simulink model "Template_v3_08_2020a"  (R2020a)
settings: Solver=FixedStepAuto  StartTime=0.0  StopTime=tsim  FixedStep=baseRate  RelTol=1e-3  EnableMultiTasking=on
values from neighbouring files (symbols this model uses):
  baseRate = 0.05    [Run_Initializer.m]
  drop_states_ARM = [ pi/2, pi/2, 0]    [Run_Initializer.m]
  drop_states_BLACK = [ xLength/2, yLength/2, 0]    [Run_Initializer.m]
  drop_states_BLUE = [ xLength/2-0.5; yLength/2; 0]    [Run_Initializer.m]
  drop_states_RED = [ xLength/2+0.5, yLength/2, pi]    [Run_Initializer.m]
  F_Black_X_nominal = 0.2196    [Run_Initializer.m]
  F_Black_Y_nominal = 0.2825    [Run_Initializer.m]
  F_Blue_X_nominal = 0.2196    [Run_Initializer.m]
  F_Blue_Y_nominal = 0.2825    [Run_Initializer.m]
  F_red_X_nominal = 0.2196    [Run_Initializer.m]
  F_red_Y_nominal = 0.2825    [Run_Initializer.m]
  F_thrusters_BLACK = [F_Black_X_nominal; F_Black_X_nominal;                             F_Black_Y_nominal; F_Black_Y_nominal; F_Black_X_nominal;                              F_Black_X_nominal; F_Black_Y_nominal; F_Black_Y_nominal]    [Run_Initializer.m]
  F_thrusters_BLUE = [F_Blue_X_nominal; F_Blue_X_nominal;                             F_Blue_Y_nominal; F_Blue_Y_nominal; F_Blue_X_nominal;                              F_Blue_X_nominal; F_Blue_Y_nominal; F_Blue_Y_nominal]    [Run_Initializer.m]
  F_thrusters_RED = [F_red_X_nominal; F_red_X_nominal;                             F_red_Y_nominal; F_red_Y_nominal; F_red_X_nominal;                              F_red_X_nominal; F_red_Y_nominal; F_red_Y_nominal]    [Run_Initializer.m]
  Gamma1 = 0.0025    [Run_Initializer.m]
  Gamma2 = 100    [Run_Initializer.m]
  Gamma3 = 10    [Run_Initializer.m]
  Gamma4 = 0.001    [Run_Initializer.m]
  Gamma5 = 100    [Run_Initializer.m]
  Gamma6 = 0.001    [Run_Initializer.m]
  home_states_BLACK = [ xLength/2; yLength/2; 0]    [Run_Initializer.m]
  home_states_BLUE = [ xLength/2-0.9; yLength/2; 0]    [Run_Initializer.m]
  home_states_RED = [ xLength/2+0.9; yLength/2; pi]    [Run_Initializer.m]
  init_states_BLACK = [ xLength/2; yLength/2; 0]    [Run_Initializer.m]
  init_states_BLUE = [ xLength/2-0.9; yLength/2; 0]    [Run_Initializer.m]
  init_states_RED = [ xLength/2+0.9; yLength/2; pi]    [Run_Initializer.m]
  Kd_elarm = 0.05    [Run_Initializer.m]
  Kd_sharm = 0.05    [Run_Initializer.m]
  Kd_tb = 0.4    [Run_Initializer.m]
  Kd_tblue = 0.4    [Run_Initializer.m]
  Kd_tr = 0.4    [Run_Initializer.m]
  Kd_wrarm = 0.005    [Run_Initializer.m]
  Kd_xb = 8    [Run_Initializer.m]
  Kd_xblue = 8    [Run_Initializer.m]
  Kd_xr = 8    [Run_Initializer.m]
  Kd_yb = 8    [Run_Initializer.m]
  Kd_yblue = 8    [Run_Initializer.m]
  Kd_yr = 8    [Run_Initializer.m]
  Kp = [0.08 0 0 ... (first row only)    [Run_Initializer.m]
  Kp_elarm = 0.08    [Run_Initializer.m]
  Kp_sharm = 0.15    [Run_Initializer.m]
  Kp_tb = 0.1    [Run_Initializer.m]
  Kp_tblue = 0.1    [Run_Initializer.m]
  Kp_tr = 0.1    [Run_Initializer.m]
  Kp_wrarm = 0.007    [Run_Initializer.m]
  Kp_xb = 2    [Run_Initializer.m]
  Kp_xblue = 2    [Run_Initializer.m]
  Kp_xr = 2    [Run_Initializer.m]
  Kp_yb = 2    [Run_Initializer.m]
  Kp_yblue = 2    [Run_Initializer.m]
  Kp_yr = 2    [Run_Initializer.m]
  Kv = [0.05 0 0 ... (first row only)    [Run_Initializer.m]
  noise_variance_BLACK = 0    [Run_Initializer.m]
  noise_variance_BLUE = 0    [Run_Initializer.m]
  noise_variance_RED = 0    [Run_Initializer.m]
  Phase0_End = Phase0_Duration    (= 10)    [Run_Initializer.m]
  Phase1_End = Phase0_Duration + Phase1_Duration    (= 15)    [Run_Initializer.m]
  Phase2_End = Phase0_Duration + Phase1_Duration +                                   Phase2_Duration    (= 35)    [Run_Initializer.m]
  Phase3_End = Phase0_Duration + Phase1_Duration +                                   Phase2_Duration + Phase3_Duration    (= 550)    [Run_Initializer.m]
  Phase3_SubPhase1_End = Phase2_End + Phase3_SubPhase1_Duration    (= 155)    [Run_Initializer.m]
  Phase3_SubPhase2_End = Phase2_End + Phase3_SubPhase1_Duration +                                   Phase3_SubPhase2_Duration    (= 165)    [Run_Initializer.m]
  Phase3_SubPhase3_End = Phase2_End + Phase3_SubPhase1_Duration +                                   Phase3_SubPhase2_Duration +                                  Phase3_SubPhase3_Duration    (= 195)    [Run_Initializer.m]
  Phase3_SubPhase4_End = Phase2_End + Phase3_SubPhase1_Duration +                                   Phase3_SubPhase2_Duration +                                  Phase3_SubPhase3_Duration +                                  Phase3_SubPhase4_Duration    [Run_Initializer.m]
  Phase4_End = Phase0_Duration + Phase1_Duration +                                   Phase2_Duration + Phase3_Duration +                                   Phase4_Duration    (= 670)    [Run_Initializer.m]
  Phase5_End = Phase0_Duration + Phase1_Duration +                                   Phase2_Duration + Phase3_Duration +                                   Phase4_Duration + Phase5_Duration    (= 690)    [Run_Initializer.m]
  thruster_dist2CG_BLACK = [83.42;-52.58;55.94;-60.05;54.08;-53.92;77.06;-55.94]    [Run_Initializer.m]
  thruster_dist2CG_BLUE = [73.54;-64.46;81.39;-60.11;64.46;-65.94;54.61;-74.39]    [Run_Initializer.m]
  thruster_dist2CG_RED = [49.92;-78.08;70.46;-63.54;81.08;-50.42;57.44;-75.96]    [Run_Initializer.m]
  Tz_lim_elarm = .1    (= 0.1)    [Run_Initializer.m]
  Tz_lim_sharm = .1    (= 0.1)    [Run_Initializer.m]
  Tz_lim_wrarm = .1    (= 0.1)    [Run_Initializer.m]
  xLength = 3.51155    [Run_Initializer.m]
  yLength = 2.41935    [Run_Initializer.m]
undefined symbols (not defined in the file or in its folder): DiscIntNeverNeededParam, model_param, platformSelection, serverRate, simMode
libraries: dspstat3 x18, raspberrypiBasiclib x10, embdlinuxlib x7, MainLibrary x6, dspsigops x6, simulink x6, mspfiltlib x3, dsparch4 x3, sensehatlib x1
(part 14 of 14)

== matlab function Template_v3_08_2020a/Phase #4: Return Home/Change RED Behavior/RED+ARM/Transpose Jacobian Controller/Transpose Generalized Jacobian /Inertia Function  ==
  data: InertiaS output; x input; model_param parameter
function InertiaS = InertiaFunc3LINK(x, model_param)
%INERTIAFUNC3LINK
%    INERTIAS = INERTIAFUNC3LINK(I0,I1,I2,I3,A1,A2,A3,B0,B1,B2,M0,M1,M2,M3,PHI,Q0,Q1,Q2,Q3)

%    This function was generated by the Symbolic Math Toolbox version 8.5.
%    15-Mar-2022 15:58:51

q0 = x(3);
q1 = x(4);
q2 = x(5);
q3 = x(6);

m0= model_param(1);                  % RED Mass
I0= model_param(2);                  % RED Inertia;
phi= model_param(7);                 % ARM Phi
b0= model_param(8);                  % ARM b0
a1= model_param(9);                  % ARM a1
b1= model_param(10);                 % ARM b1
a2= model_param(11);                 % ARM a2
b2= model_param(12);                 % ARM b2
a3= model_param(13);                 % ARM a3
b3= model_param(14);                 % ARM b3
m1= model_param(15);                 % ARM m1
m2= model_param(16);                 % ARM m2
m3= model_param(17);                 % ARM m3
I1= model_param(18);                 % ARM I1
I2= model_param(19);                 % ARM I2
I3= model_param(20);                 % ARM I3

t2 = cos(q2);
t3 = cos(q3);
t4 = a1+b1;
t5 = a2+b2;
t6 = a1.*m1;
t7 = a2.*m2;
t8 = a2.*m3;
t9 = a3.*m3;
t10 = b0.*m1;
t11 = b0.*m2;
t12 = b0.*m3;
t13 = b2.*m3;
t14 = phi+q0;
t15 = q0+q1;
t16 = q2+q3;
t17 = a1.^2;
t18 = a2.^2;
t19 = a3.^2;
t20 = b0.^2;
t21 = b1.^2;
t22 = b2.^2;
t48 = -phi;
t49 = -q1;
t50 = m0+m1+m2+m3;
t76 = a1.*b1.*m2.*2.0;
t77 = a1.*b1.*m3.*2.0;
t23 = a1.*t7;
t24 = a1.*t8;
t25 = a1.*t9;
t26 = a3.*t8;
t27 = b0.*t6;
t28 = a1.*t11;
t29 = a1.*t12;
t30 = b0.*t7;
t31 = b0.*t8;
t32 = b1.*t7;
t33 = a1.*t13;
t34 = b1.*t8;
t35 = b0.*t9;
t36 = b1.*t9;
t37 = b2.*t9;
t38 = b1.*t11;
t39 = b1.*t12;
t40 = b2.*t12;
t41 = b1.*t13;
t42 = cos(t14);
t43 = cos(t15);
t44 = cos(t16);
t45 = q2+t15;
t46 = sin(t14);
t47 = sin(t15);
t52 = t15+t16;
t54 = -t6;
t55 = -t7;
t56 = -t8;
t57 = -t9;
t58 = -t10;
t59 = -t11;
t60 = -t12;
t61 = -t13;
t62 = a1.*t6;
t63 = m2.*t17;
t64 = m3.*t17;
t65 = a2.*t7;
t66 = a2.*t8;
t67 = a3.*t9;
t69 = m2.*t21;
t70 = m3.*t21;
t71 = b2.*t13;
t81 = b2.*t8.*2.0;
t85 = m2.*t4;
t86 = m3.*t4;
t87 = m3.*t5;
t94 = phi+t49;
t95 = q1+q2+t48;
t101 = q1+t16+t48;
t106 = t10+t11+t12;
t51 = cos(t45);
t53 = sin(t45);
t68 = t67;
t72 = t23.*2.0;
t73 = t24.*2.0;
t74 = t25.*2.0;
t75 = t26.*2.0;
t78 = t32.*2.0;
t79 = t33.*2.0;
t80 = t34.*2.0;
t82 = t36.*2.0;
t83 = t37.*2.0;
t84 = t41.*2.0;
t88 = cos(t52);
t89 = -t30;
t90 = -t31;
t91 = -t35;
t92 = -t40;
t93 = sin(t52);
t96 = sin(t94);
t98 = -t85;
t99 = -t86;
t100 = -t87;
t102 = sin(t95);
t103 = t25+t36;
t104 = t26+t37;
t105 = sin(t101);
t115 = t42.*t106;
t118 = t55+t56+t61;
t119 = t58+t59+t60;
t125 = t27+t28+t29+t38+t39;
t126 = -t46.*t106;
t129 = -t43.*(t6+t85+t86);
t130 = -t47.*(t6+t85+t86);
t131 = t23+t24+t32+t33+t34+t41;
t97 = I3+t68;
t107 = t74+t82;
t108 = t75+t83;
t109 = t57.*t88;
t110 = t57.*t93;
t111 = t3.*t104;
t112 = t55+t100;
t113 = t44.*t103;
t117 = t91.*t105;
t120 = -t53.*(t7+t87);
t121 = t89+t90+t92;
t122 = -t51.*(t7+t87);
t124 = t54+t98+t99;
t127 = -t51.*(t7+t8+t13);
t128 = -t53.*(t7+t8+t13);
t133 = t2.*t131;
t134 = -t102.*(t30+t31+t40);
t135 = t96.*t125;
t136 = t72+t73+t78+t79+t80+t84;
t114 = t3.*t108;
t116 = t44.*t107;
t123 = t97+t111;
t132 = I2+t65+t66+t71+t81+t97;
t138 = t2.*t136;
t139 = t109+t127;
t140 = t110+t128;
t142 = t110+t120+t130;
t143 = t109+t122+t129;
t137 = t113+t123;
t144 = I1+t62+t63+t64+t69+t70+t76+t77+t132;
t145 = t115+t142;
t146 = t126+t143;
t147 = t113+t114+t132+t133;
t141 = t117+t137;
t148 = t117+t134+t147;
t149 = t114+t116+t117+t134+t135+t138+t144;
InertiaS = reshape([t50,0.0,t146,t143,t139,t109,0.0,t50,t145,t142,t140,t110,t146,t145,I0+t114+t116+t135.*2.0+t138+t144+b0.*t10+b0.*t11+b0.*t12-t35.*t105.*2.0-t102.*(t30.*2.0+t31.*2.0+t40.*2.0),t149,t148,t141,t143,t142,t149,t114+t116+t138+t144,t147,t137,t139,t140,t148,t147,t114+t132,t123,t109,t110,t141,t137,t123,t97],[6,6]);

end

== matlab function Template_v3_08_2020a/Phase #4: Return Home/Change RED Behavior/RED+ARM/Transpose Jacobian Controller/Transpose Generalized Jacobian /MATLAB Function ==
  data: q input; J output; InertiaS input; model_param parameter
function J  = fcn(q, InertiaS, model_param)
%#codegen

% Source: http://ieeexplore.ieee.org.proxy.library.carleton.ca/stamp/stamp.jsp?tp=&arnumber=34766
q0     = q(3);
q1     = q(4);
q2     = q(5);
q3     = q(6);

m0= model_param(1);                  % RED Mass
I0= model_param(2);                  % RED Inertia;
phi= model_param(7);                 % ARM Phi
b0= model_param(8);                  % ARM b0
a1= model_param(9);                  % ARM a1
b1= model_param(10);                 % ARM b1
a2= model_param(11);                 % ARM a2
b2= model_param(12);                 % ARM b2
a3= model_param(13);                 % ARM a3
b3= model_param(14);                 % ARM b3
m1= model_param(15);                 % ARM m1
m2= model_param(16);                 % ARM m2
m3= model_param(17);                 % ARM m3
I1= model_param(18);                 % ARM I1
I2= model_param(19);                 % ARM I2
I3= model_param(20);                 % ARM I3
l1     = a1+b1;
l2     = a2+b2;
l3     = a3+b3;

w = m0+m1+m2+m3;

% J = [ 1, 0, - l3*sin(q0 + q1 + q2 + q3) - b0*sin(phi + q0) - l1*sin(q0 + q1) - l2*sin(q0 + q1 + q2), - l3*sin(q0 + q1 + q2 + q3) - l1*sin(q0 + q1) - l2*sin(q0 + q1 + q2), - l3*sin(q0 + q1 + q2 + q3) - l2*sin(q0 + q1 + q2), -l3*sin(q0 + q1 + q2 + q3)
%       0, 1,   l3*cos(q0 + q1 + q2 + q3) + b0*cos(phi + q0) + l1*cos(q0 + q1) + l2*cos(q0 + q1 + q2),   l3*cos(q0 + q1 + q2 + q3) + l1*cos(q0 + q1) + l2*cos(q0 + q1 + q2),   l3*cos(q0 + q1 + q2 + q3) + l2*cos(q0 + q1 + q2),  l3*cos(q0 + q1 + q2 + q3)];

% Contants
K0     = m0*b0/w;
K1     = (m0*l1 + m1*b1)/w;
K2     = ((m0+m1)*l2 + m2*b2)/w;
K3     = ((m0+m1+m2)*l3 + m3*b3)/w;

% Trigonometric simplifications
s0     = sin(phi);
s1     = sin(pi/2+q1);
s2     = sin(pi/2+q1+q2);
s3     = sin(pi/2+q1+q2+q3);
c0     = cos(phi);
c1     = cos(pi/2+q1);
c2     = cos(pi/2+q1+q2);
c3     = cos(pi/2+q1+q2+q3);

% Jacobian for the base (specific)       
Jm     = [ -K1*s1-K2*s2-K3*s3 -K2*s2-K3*s3 -K3*s3 
            K1*c1+K2*c2+K3*c3  K2*c2+K3*c3  K3*c3  ];

% Jacobian for the manipulator (specific)
Js     = [ -K0*b0*s0-K1*l1*s1-K2*l2*s2-K3*l3*s3
            K0*b0*c0+K1*l1*c1+K2*l2*c2+K3*l3*c3 ];

% More constants
H      = InertiaS;
                      
Is     = H(3,3);
Im     = [H(3,4), H(3,5), H(3,6)];

% Calculate generalized Jacobian
J      = Jm - Js*(Is\Im);  

end
